simulink model "test_loop_interno_filtro_notrch"  (R2020a)
settings: Solver=VariableStepAuto  StartTime=0.0  StopTime=10.0  RelTol=1e-3
undefined symbols (not defined in the file or in its folder): denC0d, G, notch, numC0d, pi_pos
settings Model: Creator=edoar  LastModifiedBy=edoar

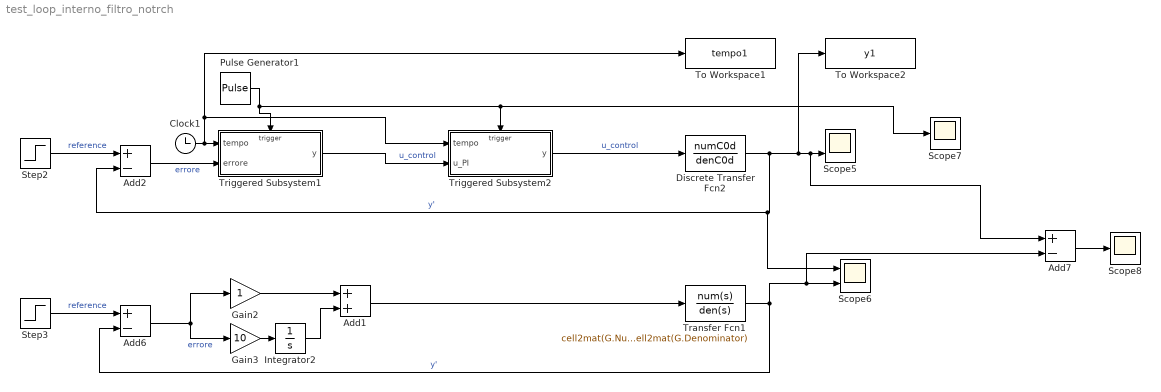
== system test_loop_interno_filtro_notrch ==
  Add1 : Sum
  Add2 : Sum  Inputs=+-
  Add6 : Sum  Inputs=+-
  Add7 : Sum  Inputs=+-
  Clock1 : Clock
  Discrete Transfer Fcn2 : DiscreteTransferFcn  Numerator=numC0d  Denominator=denC0d
  Gain2 : Gain
  Gain3 : Gain  Gain=10
  Integrator2 : Integrator
  Pulse Generator1 : DiscretePulseGenerator  PulseType=Time based  Period=0.001  PulseWidth=50
  Scope5 : Scope  NumInputPorts=2
  Scope6 : Scope  NumInputPorts=2
  Scope7 : Scope
  Scope8 : Scope
  Step2 : Step  Time=0  SampleTime=0
  Step3 : Step  Time=0  SampleTime=0
  To Workspace1 : ToWorkspace  VariableName=tempo1  SaveFormat=Timeseries  SampleTime=-1
  To Workspace2 : ToWorkspace  VariableName=y1  SaveFormat=Timeseries  SampleTime=-1
  Transfer Fcn1 : TransferFcn  Numerator=cell2mat(G.Numerator)  Denominator=cell2mat(G.Denominator)
  Triggered Subsystem1 : Subsystem  TreatAsAtomicUnit=on
  Triggered Subsystem2 : Subsystem  TreatAsAtomicUnit=on
  wires:
  Add1/1 -> Transfer Fcn1/1
  Discrete Transfer Fcn2/1 -> Add2/2, Scope6/1, Scope5/2, Add7/1, To Workspace2/1  "y'"
  Step3/1 -> Add6/1  "reference"
  Gain2/1 -> Add1/1
  Step2/1 -> Add2/1  "reference"
  Transfer Fcn1/1 -> Add6/2, Scope6/2, Add7/2  "y'"
  Pulse Generator1/1 -> Triggered Subsystem2/Trigger, Scope7/1, Triggered Subsystem1/Trigger
  Clock1/1 -> Triggered Subsystem1/1(tempo), Triggered Subsystem2/1(tempo), To Workspace1/1
  Gain3/1 -> Integrator2/1
  Integrator2/1 -> Add1/2
  Add6/1 -> Gain2/1, Gain3/1  "errore"
  Add2/1 -> Triggered Subsystem1/2(errore)  "errore"
  Add7/1 -> Scope8/1
  Triggered Subsystem1/1(y) -> Triggered Subsystem2/2(u_PI)  "u_control"
  Triggered Subsystem2/1(y) -> Discrete Transfer Fcn2/1  "u_control"

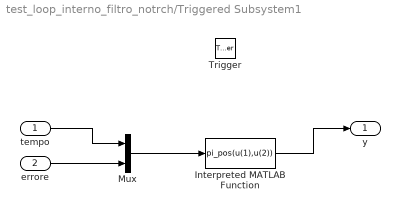
== system test_loop_interno_filtro_notrch/Triggered Subsystem1 ==
  tempo : Inport
  errore : Inport  Port=2
  Trigger : TriggerPort  VariantControl=Variant
  Interpreted MATLAB Function : MATLABFcn  MATLABFcn=pi_pos(u(1),u(2))
  Mux : Mux  Inputs=2
  y : Outport
  wires:
  Interpreted MATLAB Function/1 -> y/1
  Mux/1 -> Interpreted MATLAB Function/1
  errore/1 -> Mux/2
  tempo/1 -> Mux/1

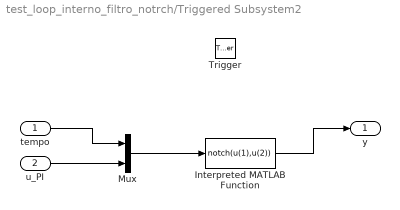
== system test_loop_interno_filtro_notrch/Triggered Subsystem2 ==
  tempo : Inport
  u_PI : Inport  Port=2
  Trigger : TriggerPort  VariantControl=Variant
  Interpreted MATLAB Function : MATLABFcn  MATLABFcn=notch(u(1),u(2))
  Mux : Mux  Inputs=2
  y : Outport
  wires:
  Interpreted MATLAB Function/1 -> y/1
  Mux/1 -> Interpreted MATLAB Function/1
  u_PI/1 -> Mux/2
  tempo/1 -> Mux/1
